simulink model "Seguidor_continuo_plantilla"  (R2016a)
settings: Solver=VariableStepAuto  StartTime=0.0  StopTime=10.0  RelTol=1e-3
values from neighbouring files (symbols this model uses):
  A = [-1,0;0,2]    [Regulador_seguidor_observador_codigo.m]
  B = [1;1]    [Regulador_seguidor_observador_codigo.m]
  C = [1,1]    [Regulador_seguidor_observador_codigo.m]
  Ki = K_dis(1:1,3:3)    [Regulador_seguidor_observador_codigo.m]
  Kp = K_dis(1:1,1:2)    [Regulador_seguidor_observador_codigo.m]
settings Model: Creator=Daniel  LastModifiedBy=Daniel

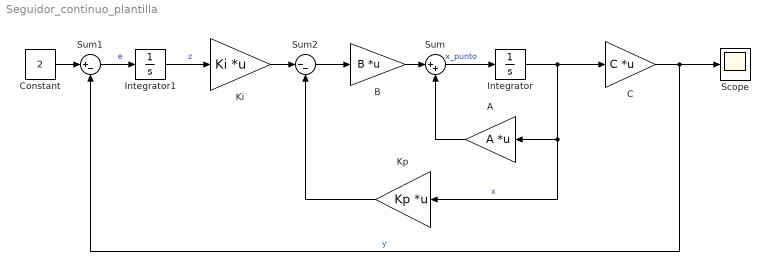
== system Seguidor_continuo_plantilla ==
  A : Gain  Gain=A  Multiplication=Matrix(K*u) (u vector)
  B : Gain  Gain=B  Multiplication=Matrix(K*u) (u vector)
  C : Gain  Gain=C  Multiplication=Matrix(K*u) (u vector)
  Constant : Constant  Value=2
  Integrator : Integrator
  Integrator1 : Integrator
  Ki : Gain  Gain=Ki  Multiplication=Matrix(K*u) (u vector)
  Kp : Gain  Gain=Kp  Multiplication=Matrix(K*u) (u vector)
  Scope : Scope
  Sum : Sum  Inputs=|++
  Sum1 : Sum  Inputs=|+-
  Sum2 : Sum  Inputs=|--
  wires:
  Integrator/1 -> Kp/1, A/1, C/1  "x"
  Sum/1 -> Integrator/1  "x_punto"
  A/1 -> Sum/2
  Integrator1/1 -> Ki/1  "z"
  Sum1/1 -> Integrator1/1  "e"
  C/1 -> Sum1/2, Scope/1  "y"
  Constant/1 -> Sum1/1
  Ki/1 -> Sum2/1
  Sum2/1 -> B/1
  B/1 -> Sum/1
  Kp/1 -> Sum2/2
